simulink model "NoLinearModel"  (R2025a)
settings: Solver=FixedStepDiscrete  StartTime=0.0  StopTime=10.0  FixedStep=SimulationStep  RelTol=1e-3
model workspace (MAT data in the model file):
  Cx = Simulink.Parameter
  Cx.Value = 1
  Cx.Complexity = 'real'
  Cx.Dimensions = [1 1]
  Cx.DataType = 'auto'
  Cy = Simulink.Parameter
  Cy.Value = 1
  Cy.Complexity = 'real'
  Cy.Dimensions = [1 1]
  Cy.DataType = 'auto'
  SimulationStep = Simulink.Parameter
  SimulationStep.Value = 0.01
  SimulationStep.Complexity = 'real'
  SimulationStep.Dimensions = [1 1]
  SimulationStep.DataType = 'auto'
  SimulationStep.DocUnits = 's'
  gravity = Simulink.Parameter
  gravity.Value = 9.81
  gravity.Complexity = 'real'
  gravity.Dimensions = [1 1]
  gravity.DataType = 'auto'
  gravity.DocUnits = 'm/s^2'
  mass = Simulink.Parameter
  mass.Value = 0.8
  mass.Complexity = 'real'
  mass.Dimensions = [1 1]
  mass.DataType = 'auto'
  mass.DocUnits = 'kg'
  pitch_K = Simulink.Parameter
  pitch_K.Value = 1
  pitch_K.Complexity = 'real'
  pitch_K.Dimensions = [1 1]
  pitch_K.DataType = 'auto'
  pitch_max = Simulink.Parameter
  pitch_max.Value = 1
  pitch_max.Complexity = 'real'
  pitch_max.Dimensions = [1 1]
  pitch_max.DataType = 'auto'
  pitch_omega = Simulink.Parameter
  pitch_omega.Value = 1
  pitch_omega.Complexity = 'real'
  pitch_omega.Dimensions = [1 1]
  pitch_omega.DataType = 'auto'
  pitch_zeta = Simulink.Parameter
  pitch_zeta.Value = 1
  pitch_zeta.Complexity = 'real'
  pitch_zeta.Dimensions = [1 1]
  pitch_zeta.DataType = 'auto'
  roll_K = Simulink.Parameter
  roll_K.Value = 1
  roll_K.Complexity = 'real'
  roll_K.Dimensions = [1 1]
  roll_K.DataType = 'auto'
  roll_max = Simulink.Parameter
  roll_max.Value = 1
  roll_max.Complexity = 'real'
  roll_max.Dimensions = [1 1]
  roll_max.DataType = 'auto'
  roll_omega = Simulink.Parameter
  roll_omega.Value = 1
  roll_omega.Complexity = 'real'
  roll_omega.Dimensions = [1 1]
  roll_omega.DataType = 'auto'
  roll_zeta = Simulink.Parameter
  roll_zeta.Value = 1
  roll_zeta.Complexity = 'real'
  roll_zeta.Dimensions = [1 1]
  roll_zeta.DataType = 'auto'
  yawp_K = Simulink.Parameter
  yawp_K.Value = 1
  yawp_K.Complexity = 'real'
  yawp_K.Dimensions = [1 1]
  yawp_K.DataType = 'auto'
  yawp_max = Simulink.Parameter
  yawp_max.Value = 1
  yawp_max.Complexity = 'real'
  yawp_max.Dimensions = [1 1]
  yawp_max.DataType = 'auto'
  yawp_tal = Simulink.Parameter
  yawp_tal.Value = 1
  yawp_tal.Complexity = 'real'
  yawp_tal.Dimensions = [1 1]
  yawp_tal.DataType = 'auto'
  zp_K = Simulink.Parameter
  zp_K.Value = 1
  zp_K.Complexity = 'real'
  zp_K.Dimensions = [1 1]
  zp_K.DataType = 'auto'
  zp_max = Simulink.Parameter
  zp_max.Value = 1
  zp_max.Complexity = 'real'
  zp_max.Dimensions = [1 1]
  zp_max.DataType = 'auto'
  zp_tal = Simulink.Parameter
  zp_tal.Value = 1
  zp_tal.Complexity = 'real'
  zp_tal.Dimensions = [1 1]
  zp_tal.DataType = 'auto'
undefined symbols (not defined in the file): DiscIntNeverNeededParam
settings Model: ParameterArgumentNames=Cx,Cy,pitch_K,pitch_max,pitch_omega,pitch_zeta,roll_K,roll_max,roll_omega,roll_zeta,yawp_K,yawp_max,yawp_tal,zp_K,zp_max,zp_tal  Creator=Gabriel Fernandes  LastModifiedBy=Gabriel Fernandes
settings OptimizationCC: DefaultParameterBehavior=Inlined  UseDivisionForNetSlopeComputation=on  GainParamInheritBuiltInType=on  UseFloatMulNetSlope=on  OptimizeBlockIOStorage=off  BufferReuse=off  ReuseModelBlockBuffer=off  GlobalBufferReuse=off  ExpressionFolding=off  EnableMemcpy=off  PassReuseOutputArgsAs=Individual arguments  LocalBlockOutputs=off  ZeroExternalMemoryAtStartup=off  ZeroInternalMemoryAtStartup=off  NoFixptDivByZeroProtection=on  EfficientFloat2IntCast=on  LifeSpan=1  OptimizeDataStoreBuffers=off  BusAssignmentInplaceUpdate=off  OptimizationLevel=level0  OptimizationCustomize=off  EfficientTunableParamExpr=on
settings DebuggingCC: ParameterTunabilityLossMsg=error
settings HardwareCC: ProdLongLongMode=on
settings SFSimCC: MATLABDynamicMemAlloc=off
settings RTWCC: SystemTargetFile=ert.tlc  PackageGeneratedCodeAndArtifacts=on  PackageName=NoLinearBuild  TemplateMakefile=ert_default_tmf  BuildConfiguration=Debug  TargetLang=C++  Description=Embedded Coder
settings CodeAppCC: ForceParamTrailComments=on  IgnoreCustomStorageClasses=off  OperatorAnnotations=on  SimulinkDataObjDesc=on  SFDataObjDesc=on  CustomSymbolStrGlobalVar=rt$N$M  CustomSymbolStrType=$N$M  CustomSymbolStrFcn=$N$M$F  CustomSymbolStrMacro=$N$M  InsertBlockDesc=on
settings ERTTargetCC: ExtModeTransport=0.0  ExtModeStaticAlloc=off  ExtModeMexFile=ext_comm  ExtModeIntrfLevel=Level1  InlinedParameterPlacement=Hierarchical  RootIOFormat=Structure reference  ERTCustomFileTemplate=example_file_process.tlc  ERTFilePackagingFormat=CompactWithDataFile  TargetLangStandard=C++11 (ISO)  GenerateSampleERTMain=on  IncludeMdlTerminateFcn=off  CombineSignalStateStructs=on  SuppressErrorStatus=on  SupportAbsoluteTime=off  CodeInterfacePackaging=C++ class  SubcomponentCodeInterfacePackaging=C++ class  SupportComplex=off

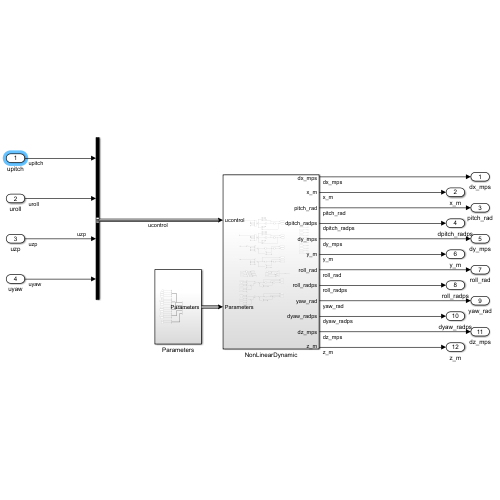
[thumbnail: Simulink's stored preview of the top-level diagram]
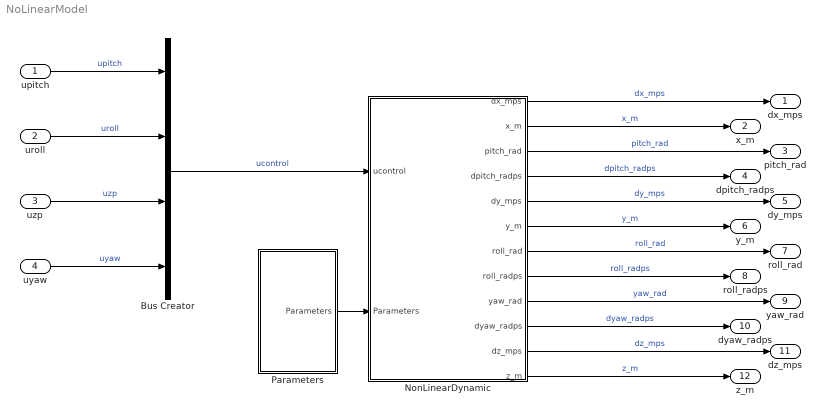
== system NoLinearModel ==
  upitch : Inport
  uroll : Inport  Port=2
  uzp : Inport  Port=3
  uyaw : Inport  Port=4
  Bus Creator : BusCreator  Inputs=4
  NonLinearDynamic : Subsystem
  Parameters : Subsystem
  dx_mps : Outport
  x_m : Outport  Port=2
  pitch_rad : Outport  Port=3
  dpitch_radps : Outport  Port=4
  dy_mps : Outport  Port=5
  y_m : Outport  Port=6
  roll_rad : Outport  Port=7
  roll_radps : Outport  Port=8
  yaw_rad : Outport  Port=9
  dyaw_radps : Outport  Port=10
  dz_mps : Outport  Port=11
  z_m : Outport  Port=12
  wires:
  NonLinearDynamic/1(dx_mps) -> dx_mps/1  "dx_mps"
  NonLinearDynamic/2(x_m) -> x_m/1  "x_m"
  NonLinearDynamic/3(pitch_rad) -> pitch_rad/1  "pitch_rad"
  NonLinearDynamic/4(dpitch_radps) -> dpitch_radps/1  "dpitch_radps"
  uyaw/1 -> Bus Creator/4  "uyaw"
  Bus Creator/1 -> NonLinearDynamic/1(ucontrol)  "ucontrol"
  uzp/1 -> Bus Creator/3  "uzp"
  uroll/1 -> Bus Creator/2  "uroll"
  upitch/1 -> Bus Creator/1  "upitch"
  Parameters/1(Parameters) -> NonLinearDynamic/2(Parameters)
  NonLinearDynamic/5(dy_mps) -> dy_mps/1  "dy_mps"
  NonLinearDynamic/7(roll_rad) -> roll_rad/1  "roll_rad"
  NonLinearDynamic/6(y_m) -> y_m/1  "y_m"
  NonLinearDynamic/8(roll_radps) -> roll_radps/1  "roll_radps"
  NonLinearDynamic/9(yaw_rad) -> yaw_rad/1  "yaw_rad"
  NonLinearDynamic/10(dyaw_radps) -> dyaw_radps/1  "dyaw_radps"
  NonLinearDynamic/11(dz_mps) -> dz_mps/1  "dz_mps"
  NonLinearDynamic/12(z_m) -> z_m/1  "z_m"

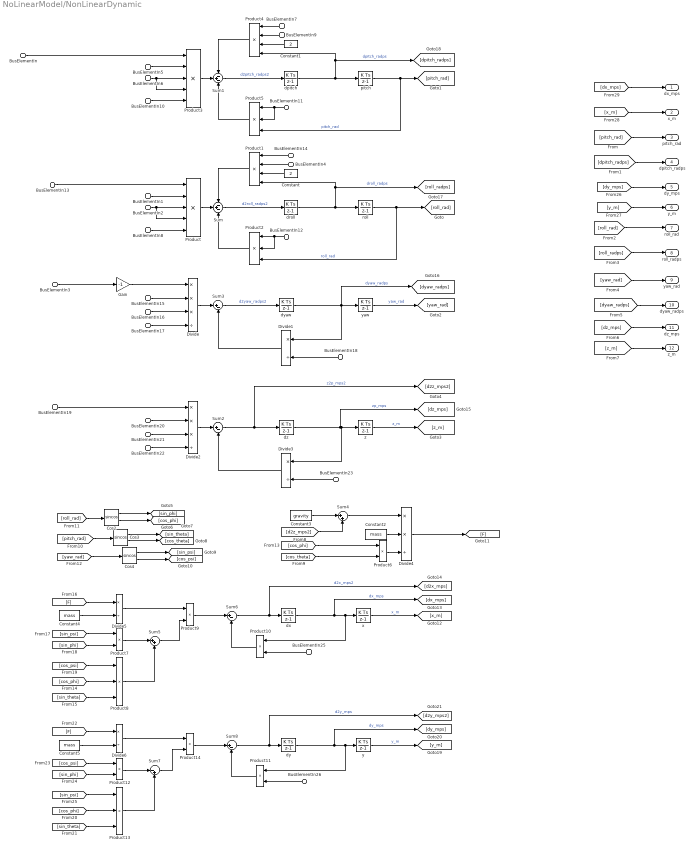
== system NoLinearModel/NonLinearDynamic ==
  BusElementIn : Inport  PortName=ucontrol  Element=upitch
  BusElementIn13 : Inport  PortName=ucontrol  Element=uroll
  BusElementIn3 : Inport  PortName=ucontrol  Element=uyaw
  BusElementIn19 : Inport  PortName=ucontrol  Element=uzp
  BusElementIn5 : Inport  Port=2  PortName=Parameters  Element=Parameterspitch.pitch_K
  BusElementIn6 : Inport  Port=2  PortName=Parameters  Element=Parameterspitch.pitch_omega
  BusElementIn9 : Inport  Port=2  PortName=Parameters  Element=Parameterspitch.pitch_omega
  BusElementIn11 : Inport  Port=2  PortName=Parameters  Element=Parameterspitch.pitch_omega
  BusElementIn7 : Inport  Port=2  PortName=Parameters  Element=Parameterspitch.pitch_zeta
  BusElementIn10 : Inport  Port=2  PortName=Parameters  Element=Parameterspitch.pitch_max
  BusElementIn1 : Inport  Port=2  PortName=Parameters  Element=Parametersroll.roll_K
  BusElementIn2 : Inport  Port=2  PortName=Parameters  Element=Parametersroll.roll_omega
  BusElementIn4 : Inport  Port=2  PortName=Parameters  Element=Parametersroll.roll_omega
  BusElementIn12 : Inport  Port=2  PortName=Parameters  Element=Parametersroll.roll_omega
  BusElementIn8 : Inport  Port=2  PortName=Parameters  Element=Parametersroll.roll_max
  BusElementIn14 : Inport  Port=2  PortName=Parameters  Element=Parametersroll.roll_zeta
  BusElementIn15 : Inport  Port=2  PortName=Parameters  Element=ParametersYawp.yawp_K
  BusElementIn16 : Inport  Port=2  PortName=Parameters  Element=ParametersYawp.yawp_max
  BusElementIn17 : Inport  Port=2  PortName=Parameters  Element=ParametersYawp.yawp_tal
  BusElementIn18 : Inport  Port=2  PortName=Parameters  Element=ParametersYawp.yawp_tal
  BusElementIn20 : Inport  Port=2  PortName=Parameters  Element=ParametersZp.zp_K
  BusElementIn21 : Inport  Port=2  PortName=Parameters  Element=ParametersZp.zp_max
  BusElementIn22 : Inport  Port=2  PortName=Parameters  Element=ParametersZp.zp_tal
  BusElementIn23 : Inport  Port=2  PortName=Parameters  Element=ParametersZp.zp_tal
  BusElementIn25 : Inport  Port=2  PortName=Parameters  Element=ParametersXY.Cx
  BusElementIn26 : Inport  Port=2  PortName=Parameters  Element=ParametersXY.Cy
  Constant : Constant  Value=2
  Constant1 : Constant  Value=2
  Constant2 : Constant  Value=mass
  Constant3 : Constant  Value=gravity
  Constant4 : Constant  Value=mass
  Constant5 : Constant  Value=mass
  Cos2 : Trigonometry  Operator=sincos
  Cos3 : Trigonometry  Operator=sincos
  Cos4 : Trigonometry  Operator=sincos
  Divide : Product  Inputs=***/
  Divide{1,3,5..6} (4 alike) : Product  Inputs=*/
  Divide2 : Product  Inputs=***/
  Divide4 : Product  Inputs=**/
  Gain : Gain  Gain=-1
  Product : Product  Inputs=5
  Product1 : Product  Inputs=4
  Product{6..7,9..12,14} (7 alike) : Product
  Product{2,5,8,13} (4 alike) : Product  Inputs=3
  Product3 : Product  Inputs=5
  Product4 : Product  Inputs=4
  Sum : Sum  Inputs=-+-
  Sum1 : Sum  Inputs=-+-
  Sum{2..3,6,8} (4 alike) : Sum  Inputs=|+-
  Sum4 : Sum  Inputs=|++
  Sum5 : Sum  Inputs=|++
  Sum7 : Sum  Inputs=|-+
  dpitch : DiscreteIntegrator  SampleTime=SimulationStep  ICPrevOutput=DiscIntNeverNeededParam  ICPrevScaledInput=DiscIntNeverNeededParam
  droll : DiscreteIntegrator  SampleTime=SimulationStep  ICPrevOutput=DiscIntNeverNeededParam  ICPrevScaledInput=DiscIntNeverNeededParam
  dx : DiscreteIntegrator  SampleTime=SimulationStep  ICPrevOutput=DiscIntNeverNeededParam  ICPrevScaledInput=DiscIntNeverNeededParam
  dy : DiscreteIntegrator  SampleTime=0.01  ICPrevOutput=DiscIntNeverNeededParam  ICPrevScaledInput=DiscIntNeverNeededParam
  dyaw : DiscreteIntegrator  SampleTime=SimulationStep  ICPrevOutput=DiscIntNeverNeededParam  ICPrevScaledInput=DiscIntNeverNeededParam
  dz : DiscreteIntegrator  SampleTime=SimulationStep  ICPrevOutput=DiscIntNeverNeededParam  ICPrevScaledInput=DiscIntNeverNeededParam
  pitch : DiscreteIntegrator  SampleTime=SimulationStep  ICPrevOutput=DiscIntNeverNeededParam  ICPrevScaledInput=DiscIntNeverNeededParam
  roll : DiscreteIntegrator  SampleTime=SimulationStep  ICPrevOutput=DiscIntNeverNeededParam  ICPrevScaledInput=DiscIntNeverNeededParam
  x : DiscreteIntegrator  SampleTime=SimulationStep  ICPrevOutput=DiscIntNeverNeededParam  ICPrevScaledInput=DiscIntNeverNeededParam
  y : DiscreteIntegrator  SampleTime=0.01  ICPrevOutput=DiscIntNeverNeededParam  ICPrevScaledInput=DiscIntNeverNeededParam
  yaw : DiscreteIntegrator  SampleTime=SimulationStep  ICPrevOutput=DiscIntNeverNeededParam  ICPrevScaledInput=DiscIntNeverNeededParam
  z : DiscreteIntegrator  SampleTime=SimulationStep  ICPrevOutput=DiscIntNeverNeededParam  ICPrevScaledInput=DiscIntNeverNeededParam
  dx_mps : Outport
  x_m : Outport  Port=2
  pitch_rad : Outport  Port=3
  dpitch_radps : Outport  Port=4
  dy_mps : Outport  Port=5
  y_m : Outport  Port=6
  roll_rad : Outport  Port=7
  roll_radps : Outport  Port=8
  yaw_rad : Outport  Port=9
  dyaw_radps : Outport  Port=10
  dz_mps : Outport  Port=11
  z_m : Outport  Port=12
  wires:
  BusElementIn/1 -> Product3/1
  BusElementIn10/1 -> Product3/5
  BusElementIn9/1 -> Product4/2
  Product3/1 -> Sum1/2
  Constant1/1 -> Product4/3
  Sum1/1 -> dpitch/1  "d2pitch_radps2"
  BusElementIn7/1 -> Product4/1
  BusElementIn6/1 -> Product3/3, Product3/4
  dpitch/1 -> pitch/1, [dpitch_radps], Product4/4  "dpitch_radps"
  BusElementIn11/1 -> Product5/2, Product5/1
  Product4/1 -> Sum1/1
  Product5/1 -> Sum1/3
  BusElementIn5/1 -> Product3/2
  pitch/1 -> [pitch_rad], Product5/3  "pitch_rad"
  [pitch_rad] -> pitch_rad/1
  [dpitch_radps] -> dpitch_radps/1
  [dx_mps] -> dx_mps/1
  [x_m] -> x_m/1
  Constant/1 -> Product1/3
  droll/1 -> roll/1, [roll_radps], Product1/4  "droll_radps"
  BusElementIn12/1 -> Product2/2, Product2/1
  BusElementIn13/1 -> Product/1
  Sum/1 -> droll/1  "d2roll_radps2"
  Product1/1 -> Sum/1
  BusElementIn1/1 -> Product/2
  roll/1 -> [roll_rad], Product2/3  "roll_rad"
  Product2/1 -> Sum/3
  BusElementIn8/1 -> Product/5
  Product/1 -> Sum/2
  BusElementIn2/1 -> Product/4, Product/3
  BusElementIn14/1 -> Product1/1
  BusElementIn4/1 -> Product1/2
  [roll_rad] -> roll_rad/1
  [roll_radps] -> roll_radps/1
  [y_m] -> y_m/1
  [dy_mps] -> dy_mps/1
  Divide/1 -> Sum3/1
  Sum3/1 -> dyaw/1  "d2yaw_radps2"
  yaw/1 -> [yaw_rad]  "yaw_rad"
  dyaw/1 -> [dyaw_radps], yaw/1, Divide1/1  "dyaw_radps"
  BusElementIn15/1 -> Divide/2
  BusElementIn3/1 -> Gain/1
  BusElementIn17/1 -> Divide/4
  Divide1/1 -> Sum3/2
  BusElementIn16/1 -> Divide/3
  BusElementIn18/1 -> Divide1/2
  [yaw_rad] -> yaw_rad/1
  [dyaw_radps] -> dyaw_radps/1
  BusElementIn21/1 -> Divide2/3
  Divide3/1 -> Sum2/2
  Sum2/1 -> [d2z_mps2], dz/1  "z2p_mps2"
  BusElementIn22/1 -> Divide2/4
  dz/1 -> [dz_mps], z/1, Divide3/1  "zp_mps"
  Divide2/1 -> Sum2/1
  z/1 -> [z_m]  "z_m"
  BusElementIn20/1 -> Divide2/2
  BusElementIn19/1 -> Divide2/1
  BusElementIn23/1 -> Divide3/2
  [dz_mps] -> dz_mps/1
  [z_m] -> z_m/1
  Constant3/1 -> Sum4/1
  [yaw_rad] -> Cos4/1
  Cos3/2 -> [cos_theta]
  [cos_theta] -> Product6/2
  [cos_phi] -> Product6/1
  [d2z_mps2] -> Sum4/2
  Sum4/1 -> Divide4/1
  [roll_rad] -> Cos2/1
  Cos2/1 -> [sin_phi]
  [pitch_rad] -> Cos3/1
  Product6/1 -> Divide4/3
  Cos4/2 -> [cos_psi]
  Divide4/1 -> [F]
  Cos2/2 -> [cos_phi]
  Cos4/1 -> [sin_psi]
  Constant2/1 -> Divide4/2
  Cos3/1 -> [sin_theta]
  Divide5/1 -> Product9/1
  [cos_psi] -> Product8/1
  dx/1 -> [dx_mps], x/1, Product10/1  "dx_mps"
  [cos_phi] -> Product8/2
  [sin_theta] -> Product8/3
  BusElementIn25/1 -> Product10/2
  Sum5/1 -> Product9/2
  Constant4/1 -> Divide5/2
  Product8/1 -> Sum5/2
  [sin_phi] -> Product7/2
  Product10/1 -> Sum6/2
  Sum6/1 -> [d2x_mps], dx/1  "d2x_mps2"
  Product7/1 -> Sum5/1
  Product9/1 -> Sum6/1
  [F] -> Divide5/1
  [sin_psi] -> Product7/1
  x/1 -> [x_m]  "x_m"
  Sum7/1 -> Product14/2
  y/1 -> [y_m]  "y_m"
  BusElementIn26/1 -> Product11/2
  Divide6/1 -> Product14/1
  Product14/1 -> Sum8/1
  [cos_psi] -> Product12/1
  Product11/1 -> Sum8/2
  [sin_psi] -> Product13/1
  [sin_theta] -> Product13/3
  [F] -> Divide6/1
  Constant5/1 -> Divide6/2
  [cos_phi] -> Product13/2
  [sin_phi] -> Product12/2
  Product13/1 -> Sum7/2
  dy/1 -> [dy_mps], y/1, Product11/1  "dy_mps"
  Product12/1 -> Sum7/1
  Sum8/1 -> [d2y_mps2], dy/1  "d2y_mps"
  Gain/1 -> Divide/1

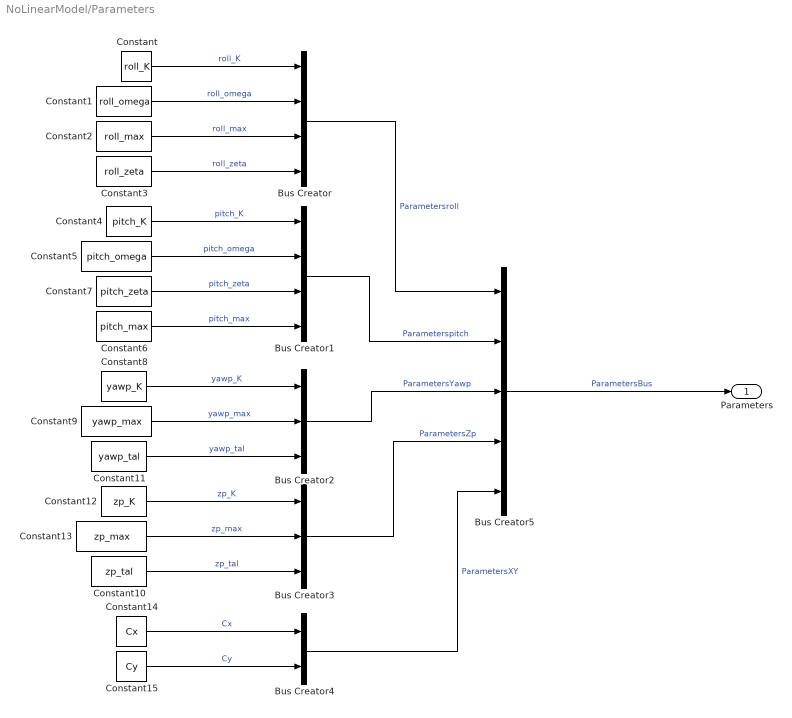
== system NoLinearModel/Parameters ==
  Bus Creator : BusCreator  Inputs=4
  Bus Creator1 : BusCreator  Inputs=4
  Bus Creator2 : BusCreator  Inputs=3
  Bus Creator3 : BusCreator  Inputs=3
  Bus Creator4 : BusCreator  Inputs=2
  Bus Creator5 : BusCreator  Inputs=5
  Constant : Constant  Value=roll_K
  Constant1 : Constant  Value=roll_omega
  Constant10 : Constant  Value=zp_tal
  Constant11 : Constant  Value=yawp_tal
  Constant12 : Constant  Value=zp_K
  Constant13 : Constant  Value=zp_max
  Constant14 : Constant  Value=Cx
  Constant15 : Constant  Value=Cy
  Constant2 : Constant  Value=roll_max
  Constant3 : Constant  Value=roll_zeta
  Constant4 : Constant  Value=pitch_K
  Constant5 : Constant  Value=pitch_omega
  Constant6 : Constant  Value=pitch_max
  Constant7 : Constant  Value=pitch_zeta
  Constant8 : Constant  Value=yawp_K
  Constant9 : Constant  Value=yawp_max
  Parameters : Outport
  wires:
  Constant3/1 -> Bus Creator/4  "roll_zeta"
  Constant12/1 -> Bus Creator3/1  "zp_K"
  Bus Creator4/1 -> Bus Creator5/5  "ParametersXY"
  Constant7/1 -> Bus Creator1/3  "pitch_zeta"
  Constant14/1 -> Bus Creator4/1  "Cx"
  Constant5/1 -> Bus Creator1/2  "pitch_omega"
  Constant/1 -> Bus Creator/1  "roll_K"
  Bus Creator1/1 -> Bus Creator5/2  "Parameterspitch"
  Constant2/1 -> Bus Creator/3  "roll_max"
  Constant4/1 -> Bus Creator1/1  "pitch_K"
  Constant9/1 -> Bus Creator2/2  "yawp_max"
  Constant10/1 -> Bus Creator3/3  "zp_tal"
  Bus Creator2/1 -> Bus Creator5/3  "ParametersYawp"
  Bus Creator3/1 -> Bus Creator5/4  "ParametersZp"
  Constant13/1 -> Bus Creator3/2  "zp_max"
  Constant11/1 -> Bus Creator2/3  "yawp_tal"
  Constant8/1 -> Bus Creator2/1  "yawp_K"
  Constant1/1 -> Bus Creator/2  "roll_omega"
  Bus Creator5/1 -> Parameters/1  "ParametersBus"
  Constant6/1 -> Bus Creator1/4  "pitch_max"
  Constant15/1 -> Bus Creator4/2  "Cy"
  Bus Creator/1 -> Bus Creator5/1  "Parametersroll"
